simulink model "drive_elastically_coupled"  (R2024b)
settings: Solver=FixedStepAuto  StartTime=0.0  StopTime=80  FixedStep=0.0001  RelTol=1e-3
values from neighbouring files (symbols this model uses):
  C_E = 5.9898    [motor_init.m]
  C_M = 0.778    [motor_init.m]
  c_welle = 5    [flex_welle_init.m]    (also in star_welle_init.m = 900)
  d_welle = 0.1    [flex_welle_init.m]    (also in star_welle_init.m)
  Kb1ia = 15    [ad_hoc_param.m]    (also in opt_motor_BO_SO.m = Kb1; opt_motorlast_BO_SO.m = Kb1)
  Kb1pa = 15    [ad_hoc_param.m]    (also in opt_motor_BO_SO.m = Tb1*Kb1; opt_motorlast_BO_SO.m = Tb1*Kb1)
  Ks2ia = 3    [ad_hoc_param.m]    (also in opt_motor_BO_SO.m = Ks2; opt_motorlast_BO_SO.m = Ks2)
  Ks2pa = 3    [ad_hoc_param.m]    (also in opt_motor_BO_SO.m = Ts2*Ks2; opt_motorlast_BO_SO.m = Ts2*Ks2)
  L_A = 0.05    [motor_init.m]
  R_A = 11.3    [motor_init.m]
  R_E = 1    [motor_init.m]
  T_E = 1    [motor_init.m]
  Tf = 0.05    [motor_init.m]    (also in opt_motor_BO_SO.m; opt_motorlast_BO_SO.m)
  thetaA = 1    [flex_welle_init.m]    (also in star_welle_init.m)
  thetaM = 0.1    [flex_welle_init.m]    (also in motor_init.m; star_welle_init.m)
  Ttot = 0.003    [motor_init.m]
libraries: simulink x2
settings Model: Creator=aviehweider  LastModifiedBy=aviehweider
settings RTWCC: GPUComputeCapability=3.5

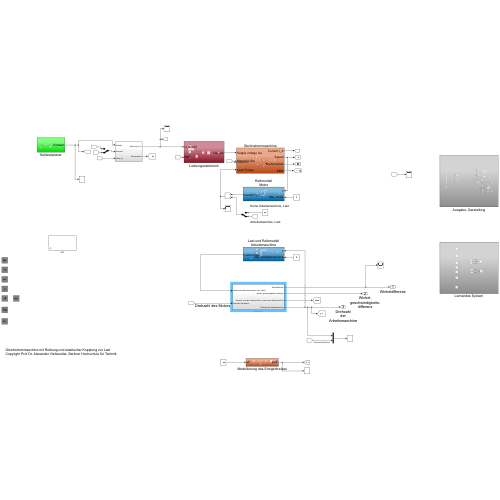
[thumbnail: Simulink's stored preview of the top-level diagram]
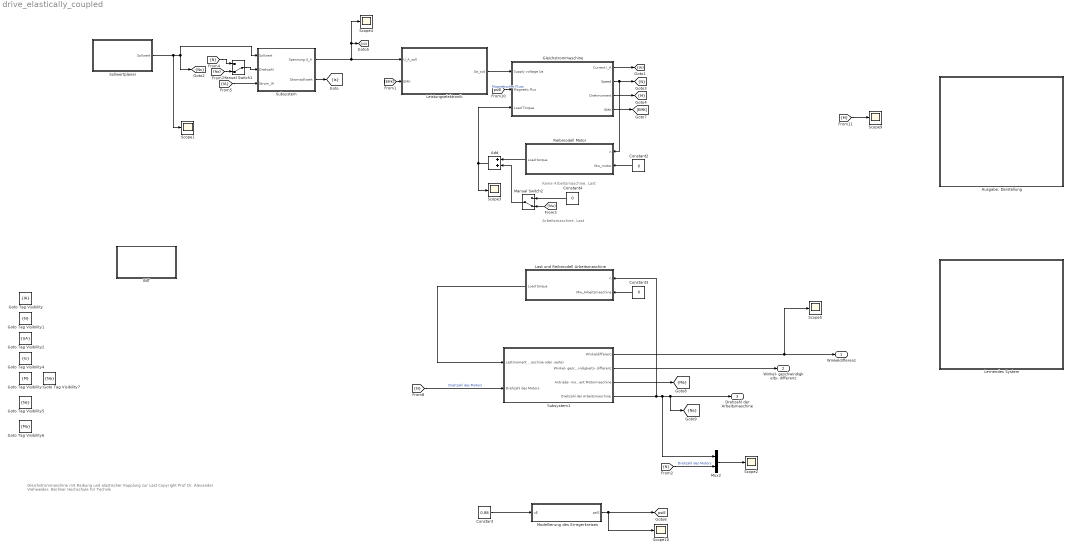
== system drive_elastically_coupled ==
  note: Gleichstrommaschine mit Reibung und elastischer Kopplung zur Last
      | Copyright Prof Dr. Alexander Viehweider, Berliner Hochschule für Technik
  note: Keine Arbeitsmaschine, Last
  note: Arbeitsmaschine, Last
  Add : Sum
  "Ausgabe, Darstellung" : Subsystem
  Constant : Constant  Value=0.88
  Constant2 : Constant  Value=0
  Constant3 : Constant  Value=0
  Constant4 : Constant  Value=0
  Gleichstrommaschine : Subsystem
  Goto Tag Visibility : GotoTagVisibility  GotoTag=IA
  Goto Tag Visibility1 : GotoTagVisibility  GotoTag=N
  Goto Tag Visibility2 : GotoTagVisibility  GotoTag=UA
  Goto Tag Visibility3 : GotoTagVisibility  GotoTag=M
  Goto Tag Visibility4 : GotoTagVisibility  GotoTag=Is
  Goto Tag Visibility5 : GotoTagVisibility  GotoTag=Ns
  Goto Tag Visibility6 : GotoTagVisibility  GotoTag=Ma
  Goto Tag Visibility7 : GotoTagVisibility  GotoTag=Na
  INIT : Subsystem
      mask DialogControl Control2 Prompt: gnm_init
  Last und Reibmodell Arbeitsmaschine : Subsystem
  Leistungselektronik : Subsystem
  Lernendes System : Subsystem
  Manual Switch1 : ManualSwitch  CurrentSetting=0
  Manual Switch2 : ManualSwitch  CurrentSetting=0
  Modellierung des Erregerkreises : Subsystem
  Mux2 : Mux  Inputs=2
  Reibmodell Motor : Subsystem
  Scope{1..5,9..10} (7 alike) : Scope
  Sollwertplaner : Subsystem
  Subsystem : Subsystem
  Subsystem1 : Subsystem
  Winkeldifferenz : Outport
  Winkel- geschwindigkeits- differenz : Outport  Port=2
  Drehzahl der Arbeitsmaschine : Outport  Port=3
  tag scope: IA=scoped, Is=scoped, M=scoped, Ma=scoped, N=scoped, Na=scoped, Ns=scoped, UA=scoped, psiE=global
  wires:
  [psiE] -> Gleichstrommaschine/2(Magnetic flux)  "Magnetischer Fluss"
  Subsystem/2(Stromsollwert) -> [Is]
  Gleichstrommaschine/1(Current I_A) -> [IA]
  Gleichstrommaschine/2(Speed) -> Reibmodell Motor/1(n), [N]
  [IA] -> Subsystem/3(Strom_IA)
  Gleichstrommaschine/3(Drehmoment) -> [M]
  Sollwertplaner/1(Sollwert) -> Scope1/1, Subsystem/1(Sollwert), [Ns]
  Modellierung des Erregerkreises/1(psiE) -> Scope10/1, [psiE]
  Constant/1 -> Modellierung des Erregerkreises/1(uE)
  [M] -> Scope9/1
  Subsystem/1(Spannung U_A) -> Scope4/1, [UA], Leistungselektronik/1(U_A_soll)
  Leistungselektronik/1(Ua_out) -> Gleichstrommaschine/1(Supply voltage Ua)
  Gleichstrommaschine/4(EMK) -> [EMK]
  [EMK] -> Leistungselektronik/2(EMK)
  [N] -> Subsystem1/2(Drehzahl des Motors)  "Drehzahl des Motors"
  Subsystem1/3(Antriebs- moment Lastmaschine= Lastmoment Motormaschine) -> [Ma]
  Subsystem1/1(Winkeldifferenz) -> Scope5/1, Winkeldifferenz/1
  Subsystem1/4(Drehzahl der Arbeitsmaschine) -> Last und Reibmodell Arbeitsmaschine/1(n), Mux2/1, [Na], Drehzahl der Arbeitsmaschine/1
  Subsystem1/2(Winkel- geschwindigkeits- differenz) -> Winkel- geschwindigkeits- differenz/1
  Mux2/1 -> Scope2/1
  [N] -> Mux2/2  "Drehzahl des Motors"
  Constant2/1 -> Reibmodell Motor/2(Mw_motor)
  Constant3/1 -> Last und Reibmodell Arbeitsmaschine/2(Mw_Arbeitsmaschine)
  Reibmodell Motor/1(Load torque) -> Add/1
  [Ma] -> Manual Switch2/2
  Manual Switch2/1 -> Add/2
  Add/1 -> Scope3/1, Gleichstrommaschine/3(Load Torque)
  Constant4/1 -> Manual Switch2/1
  Last und Reibmodell Arbeitsmaschine/1(Load torque) -> Subsystem1/1(Lastmoment Arbeits(maschine oder -seite))
  [Na] -> Manual Switch1/2
  Manual Switch1/1 -> Subsystem/2(Drehzahl)
  [N] -> Manual Switch1/1

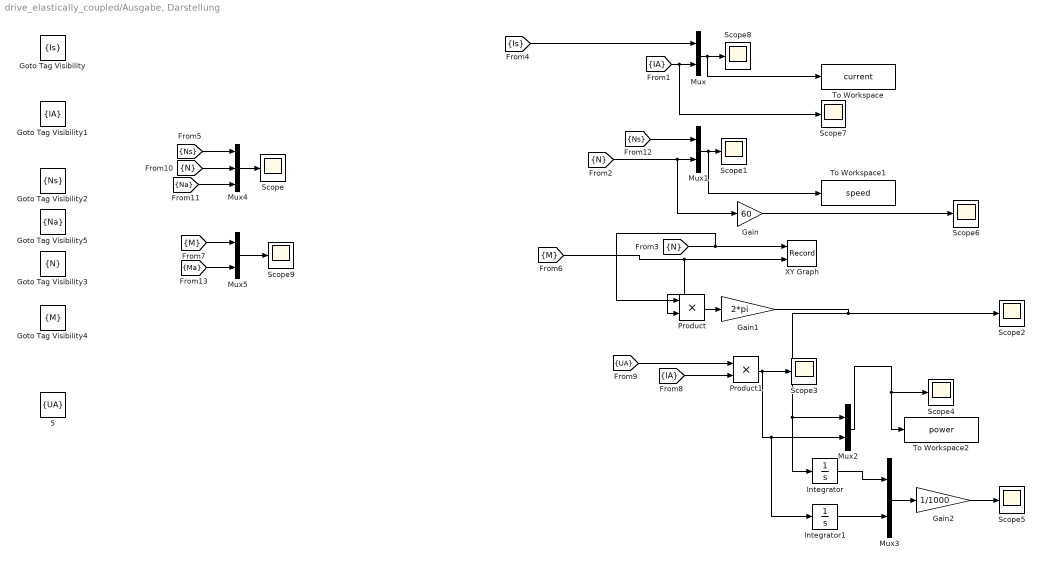
== system drive_elastically_coupled/Ausgabe, Darstellung ==
  5 : GotoTagVisibility  GotoTag=UA
  Gain : Gain  Gain=60
  Gain1 : Gain  Gain=2*pi
  Gain2 : Gain  Gain=1/1000
  Goto Tag Visibility : GotoTagVisibility  GotoTag=Is
  Goto Tag Visibility1 : GotoTagVisibility  GotoTag=IA
  Goto Tag Visibility2 : GotoTagVisibility  GotoTag=Ns
  Goto Tag Visibility3 : GotoTagVisibility  GotoTag=N
  Goto Tag Visibility4 : GotoTagVisibility  GotoTag=M
  Goto Tag Visibility5 : GotoTagVisibility  GotoTag=Na
  Integrator : Integrator
  Integrator1 : Integrator
  Mux{,1..3,5} (5 alike) : Mux  Inputs=2
  Mux4 : Mux  Inputs=3
  Product : Product
  Product1 : Product
  Scope{,1..9} (10 alike) : Scope
  To Workspace : ToWorkspace  VariableName=current  SaveFormat=Structure  SampleTime=-1
  To Workspace1 : ToWorkspace  VariableName=speed  SaveFormat=Structure  SampleTime=-1
  To Workspace2 : ToWorkspace  VariableName=power  SaveFormat=Structure  SampleTime=-1
  XY Graph : Record  FileSettingsInternal="{\"entries\":[{\"content\":{\"excelSettings\":{\"content\":{},\"type\":\"Streamout.ExcelSettings\"}},\"type\":\"Streamout.FileSettingStorage\",\"uuid\":\"\"}],\"packageUris\":[\"http:\\/\\/schema.mathworks.com\\/mf0\\/streamout_blocks\\/R2020a\"],\"version\":\"1.0\"}"  Layout=[1 1]  SignalsInternal="{\"entries\":[{\"content\":{\"signals\":[{\"content\":{\"blockPath\":[],\"dimensions\":[1],\"domain\":\"\",\"lineColor\":\"#fe330a\",\"lineWidth\":2,\"port\":1,\"signalID\":1,\"signalName\":\"From3\"},\"type\":\"RecordBlkView.Signal\",\"uuid\":\"\"},{\"content\":{\"blockPath\":[],\"dimensions\":[1],\"domain\":\"\",\"lineColor\":\"#22b573\",\"lineWidth\":2,\"port\":2,\"signalID\":2,\"signalName\":\"From6\"},\"type\":\"RecordBlkView.Signal\",\"uuid\":\"\"}]},\"type\":\"RecordBlkView.InputSignals\",\"uuid\":\"\"}],\"packageUris\":[\"http:\\/\\/schema.mathworks.com\\/mf0\\/streamout_blocks\\/R2020a\"],\"version\":\"1.0\"}"  VisualizationBindings="{\"xyplotplugin\":{\"info\":[{\"series\":[],\"subplotID\":1}]}}"  CompatibilityTag=XY
  wires:
  [N] -> Product/1, XY Graph/1
  [Ns] -> Mux1/1
  [N] -> Gain/1, Mux1/2
  Product1/1 -> Scope3/1, Integrator1/1, Mux2/2
  [UA] -> Product1/1
  [M] -> Product/2, XY Graph/2
  [Is] -> Mux/1
  Mux2/1 -> Scope4/1, To Workspace2/1
  Gain1/1 -> Scope2/1, Mux2/1, Integrator/1
  Mux/1 -> Scope8/1, To Workspace/1
  Mux1/1 -> Scope1/1, To Workspace1/1
  [IA] -> Scope7/1, Mux/2
  Integrator1/1 -> Mux3/2
  [IA] -> Product1/2
  Mux3/1 -> Gain2/1
  Product/1 -> Gain1/1
  Integrator/1 -> Mux3/1
  Gain/1 -> Scope6/1
  Gain2/1 -> Scope5/1
  [N] -> Mux4/2
  [Ns] -> Mux4/1
  Mux4/1 -> Scope/1
  [Na] -> Mux4/3
  Mux5/1 -> Scope9/1
  [M] -> Mux5/1
  [Ma] -> Mux5/2

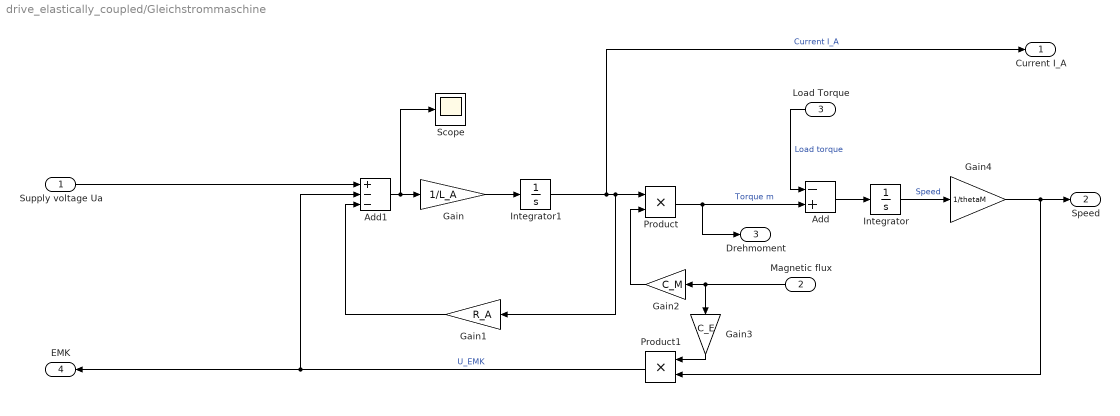
== system drive_elastically_coupled/Gleichstrommaschine ==
  Supply voltage Ua : Inport
  Magnetic flux : Inport  Port=2
  Load Torque : Inport  Port=3
  Add : Sum  Inputs=-+
  Add1 : Sum  Inputs=+--
  Gain : Gain  Gain=1/L_A
  Gain1 : Gain  Gain=R_A
  Gain2 : Gain  Gain=C_M
  Gain3 : Gain  Gain=C_E
  Gain4 : Gain  Gain=1/thetaM
  Integrator : Integrator
  Integrator1 : Integrator
  Product : Product
  Product1 : Product
  Scope : Scope
  Current I_A : Outport
  Speed : Outport  Port=2
  Drehmoment : Outport  Port=3
  EMK : Outport  Port=4
  wires:
  Integrator/1 -> Gain4/1  "Speed"
  Product/1 -> Drehmoment/1, Add/2  "Torque m"
  Add/1 -> Integrator/1
  Integrator1/1 -> Current I_A/1, Gain1/1, Product/1  "Current I_A"
  Product1/1 -> EMK/1, Add1/2  "U_EMK"
  Gain1/1 -> Add1/3
  Add1/1 -> Scope/1, Gain/1
  Magnetic flux/1 -> Gain2/1, Gain3/1
  Gain/1 -> Integrator1/1
  Load Torque/1 -> Add/1  "Load torque"
  Supply voltage Ua/1 -> Add1/1
  Gain2/1 -> Product/2
  Gain3/1 -> Product1/1
  Gain4/1 -> Product1/2, Speed/1

== system drive_elastically_coupled/INIT ==

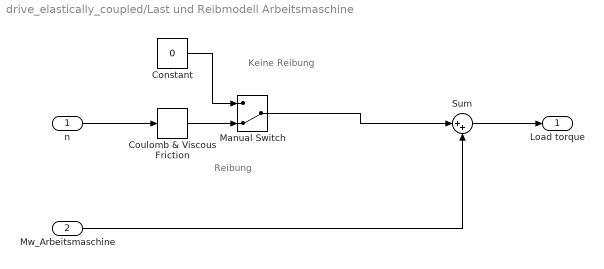
== system drive_elastically_coupled/Last und Reibmodell Arbeitsmaschine ==
  note: Keine Reibung
  note: Reibung
  n : Inport
  Mw_Arbeitsmaschine : Inport  Port=2
  Constant : Constant  Value=0
  Coulomb & Viscous Friction : simulink/Discontinuities/Coulomb & Viscous Friction  offset=[0.05]  gain=0.1
  Manual Switch : ManualSwitch  CurrentSetting=0
  Sum : Sum  Inputs=|++
  Load torque : Outport
  wires:
  n/1 -> Coulomb & Viscous Friction/1
  Mw_Arbeitsmaschine/1 -> Sum/2
  Sum/1 -> Load torque/1
  Coulomb & Viscous Friction/1 -> Manual Switch/2
  Manual Switch/1 -> Sum/1
  Constant/1 -> Manual Switch/1

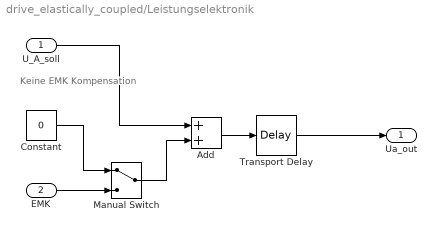
== system drive_elastically_coupled/Leistungselektronik ==
  note: Keine EMK Kompensation
  U_A_soll : Inport
  EMK : Inport  Port=2
  Add : Sum
  Constant : Constant  Value=0
  Manual Switch : ManualSwitch
  Transport Delay : TransportDelay  DelayTime=Ttot
  Ua_out : Outport
  wires:
  Transport Delay/1 -> Ua_out/1
  U_A_soll/1 -> Add/1
  Add/1 -> Transport Delay/1
  EMK/1 -> Manual Switch/2
  Manual Switch/1 -> Add/2
  Constant/1 -> Manual Switch/1

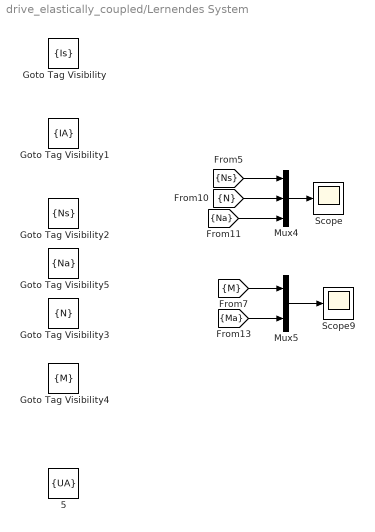
== system drive_elastically_coupled/Lernendes System ==
  5 : GotoTagVisibility  GotoTag=UA
  Goto Tag Visibility : GotoTagVisibility  GotoTag=Is
  Goto Tag Visibility1 : GotoTagVisibility  GotoTag=IA
  Goto Tag Visibility2 : GotoTagVisibility  GotoTag=Ns
  Goto Tag Visibility3 : GotoTagVisibility  GotoTag=N
  Goto Tag Visibility4 : GotoTagVisibility  GotoTag=M
  Goto Tag Visibility5 : GotoTagVisibility  GotoTag=Na
  Mux4 : Mux  Inputs=3
  Mux5 : Mux  Inputs=2
  Scope : Scope
  Scope9 : Scope
  wires:
  [N] -> Mux4/2
  [Ns] -> Mux4/1
  Mux4/1 -> Scope/1
  [Na] -> Mux4/3
  Mux5/1 -> Scope9/1
  [M] -> Mux5/1
  [Ma] -> Mux5/2

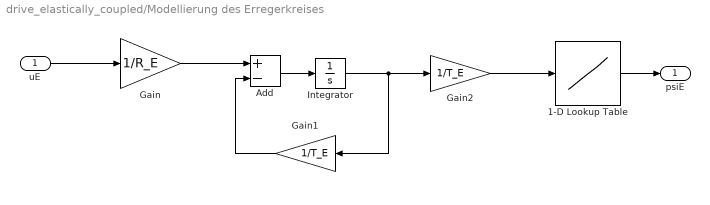
== system drive_elastically_coupled/Modellierung des Erregerkreises ==
  uE : Inport
  1-D Lookup Table : Lookup_n-D  NumberOfTableDimensions=1  BreakpointsForDimension1=[-5:5]  Table=1.5*tanh([-5:5])  InternalRulePriority=Speed  RndMeth=Simplest
  Add : Sum  Inputs=+-
  Gain : Gain  Gain=1/R_E
  Gain1 : Gain  Gain=1/T_E
  Gain2 : Gain  Gain=1/T_E
  Integrator : Integrator  InitialCondition=0.88
  psiE : Outport
  wires:
  uE/1 -> Gain/1
  Gain/1 -> Add/1
  Integrator/1 -> Gain1/1, Gain2/1
  1-D Lookup Table/1 -> psiE/1
  Add/1 -> Integrator/1
  Gain1/1 -> Add/2
  Gain2/1 -> 1-D Lookup Table/1

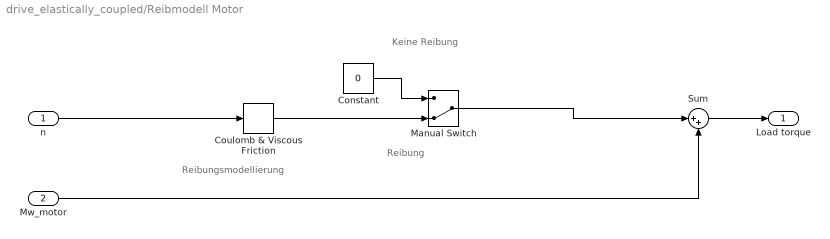
== system drive_elastically_coupled/Reibmodell Motor ==
  note: Reibungsmodellierung
  note: Reibung
  note: Keine Reibung
  n : Inport
  Mw_motor : Inport  Port=2
  Constant : Constant  Value=0
  Coulomb & Viscous Friction : simulink/Discontinuities/Coulomb & Viscous Friction  offset=0.025  gain=0.05
  Manual Switch : ManualSwitch  CurrentSetting=0
  Sum : Sum  Inputs=|++
  Load torque : Outport
  wires:
  n/1 -> Coulomb & Viscous Friction/1
  Sum/1 -> Load torque/1
  Mw_motor/1 -> Sum/2
  Coulomb & Viscous Friction/1 -> Manual Switch/2
  Manual Switch/1 -> Sum/1
  Constant/1 -> Manual Switch/1

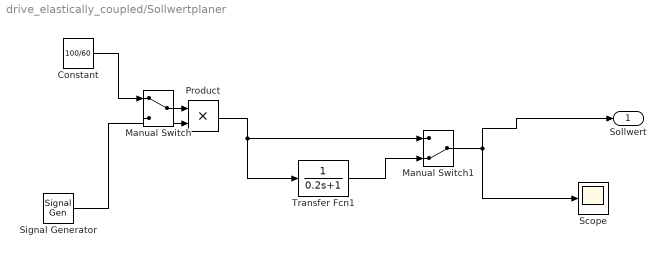
== system drive_elastically_coupled/Sollwertplaner ==
  Constant : Constant  Value=100/60
  Manual Switch : ManualSwitch
  Manual Switch1 : ManualSwitch  CurrentSetting=0
  Product : Product
  Scope : Scope
  Signal Generator : SignalGenerator  WaveForm=square  Amplitude=-1  Frequency=0.05
  Transfer Fcn1 : TransferFcn  Denominator=[0.2 1]
  Sollwert : Outport
  wires:
  ? -> Manual Switch/2  "Sollwert"
  Constant/1 -> Manual Switch/1
  Manual Switch/1 -> Product/1
  Signal Generator/1 -> Product/2
  Product/1 -> Manual Switch1/1, Transfer Fcn1/1
  Manual Switch1/1 -> Sollwert/1, Scope/1
  Transfer Fcn1/1 -> Manual Switch1/2

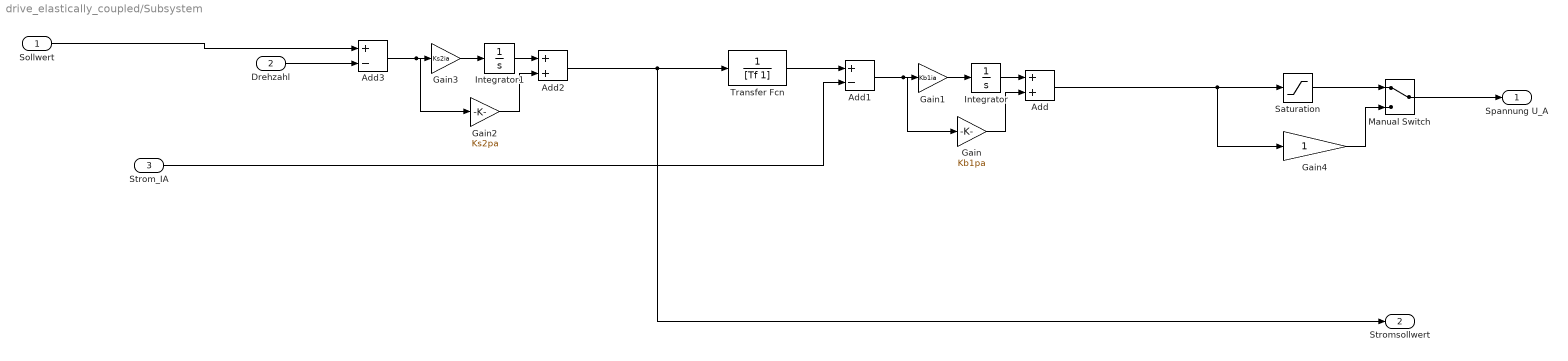
== system drive_elastically_coupled/Subsystem ==
  Sollwert : Inport
  Drehzahl : Inport  Port=2
  Strom_IA : Inport  Port=3
  Add : Sum
  Add1 : Sum  Inputs=+-
  Add2 : Sum
  Add3 : Sum  Inputs=+-
  Gain : Gain  Gain=Kb1pa
  Gain1 : Gain  Gain=Kb1ia
  Gain2 : Gain  Gain=Ks2pa
  Gain3 : Gain  Gain=Ks2ia
  Gain4 : Gain
  Integrator : Integrator
  Integrator1 : Integrator
  Manual Switch : ManualSwitch
  Saturation : Saturate  UpperLimit=400  LowerLimit=-400
  Transfer Fcn : TransferFcn  Denominator=[Tf 1]
  Spannung U_A : Outport
  Stromsollwert : Outport  Port=2
  wires:
  Manual Switch/1 -> Spannung U_A/1
  Add2/1 -> Transfer Fcn/1, Stromsollwert/1
  Strom_IA/1 -> Add1/2
  Drehzahl/1 -> Add3/2
  Gain4/1 -> Manual Switch/2
  Gain3/1 -> Integrator1/1
  Saturation/1 -> Manual Switch/1
  Transfer Fcn/1 -> Add1/1
  Add/1 -> Gain4/1, Saturation/1
  Sollwert/1 -> Add3/1
  Gain1/1 -> Integrator/1
  Gain2/1 -> Add2/2
  Add1/1 -> Gain1/1, Gain/1
  Gain/1 -> Add/2
  Integrator1/1 -> Add2/1
  Add3/1 -> Gain3/1, Gain2/1
  Integrator/1 -> Add/1

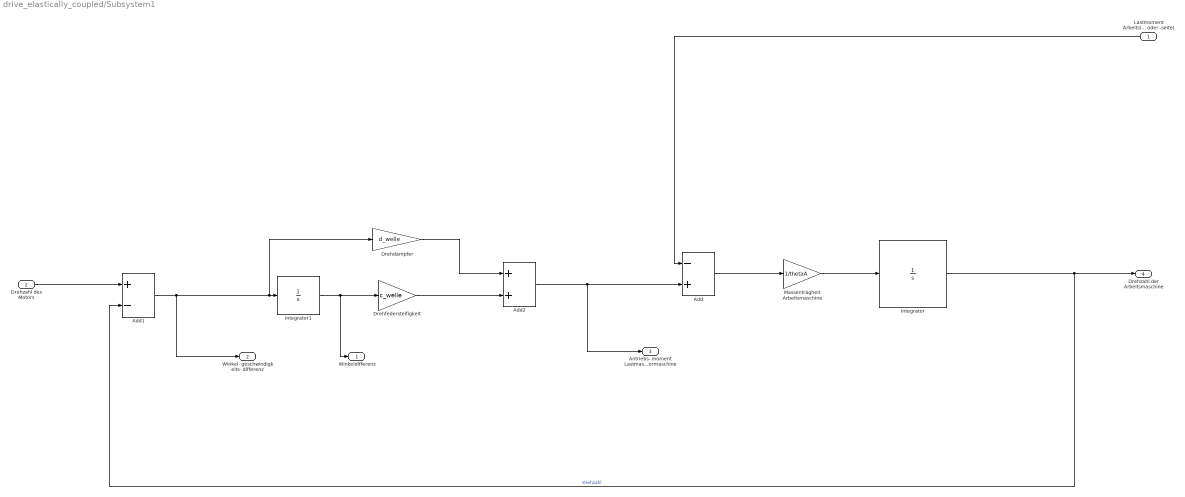
== system drive_elastically_coupled/Subsystem1 ==
  Lastmoment Arbeits(maschine oder -seite) : Inport
  Drehzahl des Motors : Inport  Port=2
  Add : Sum  Inputs=-+
  Add1 : Sum  Inputs=+-
  Add2 : Sum
  Drehdämpfer : Gain  Gain=d_welle
  Drehfedersteifigkeit : Gain  Gain=c_welle
  Integrator : Integrator
  Integrator1 : Integrator
  Massenträgheit Arbeitsmaschine : Gain  Gain=1/thetaA
  Winkeldifferenz : Outport
  Winkel- geschwindigkeits- differenz : Outport  Port=2
  Antriebs- moment Lastmaschine= Lastmoment Motormaschine : Outport  Port=3
  Drehzahl der Arbeitsmaschine : Outport  Port=4
  wires:
  Add2/1 -> Antriebs- moment Lastmaschine= Lastmoment Motormaschine/1, Add/2
  Add1/1 -> Winkel- geschwindigkeits- differenz/1, Drehdämpfer/1, Integrator1/1
  Integrator/1 -> Drehzahl der Arbeitsmaschine/1, Add1/2  "Drehzahl"
  Drehfedersteifigkeit/1 -> Add2/2
  Massenträgheit Arbeitsmaschine/1 -> Integrator/1
  Drehdämpfer/1 -> Add2/1
  Integrator1/1 -> Winkeldifferenz/1, Drehfedersteifigkeit/1
  Add/1 -> Massenträgheit Arbeitsmaschine/1
  Drehzahl des Motors/1 -> Add1/1
  Lastmoment Arbeits(maschine oder -seite)/1 -> Add/1
